simulink model "powertrain"  (R2026a)
settings: Solver=VariableStepAuto  StopTime=0.5  FixedStep=1/20e3  MaxStep=1e-5
PreLoadFcn:
  | try, p = fileparts(which(bdroot)); addpath(fullfile(p,'..', 'scripts')); addpath(fullfile(p,'..', 'models')); addpath(p); catch, end; init;
InitFcn:
  | try, p = fileparts(which(bdroot)); addpath(fullfile(p,'..', 'scripts')); addpath(fullfile(p,'..', 'models')); addpath(p); catch, end; init;
libraries: mcbcontrolslib x1
settings Model: Creator=probst  LastModifiedBy=niklasprobst
settings DebuggingCC: ParameterPrecisionLossMsg=none

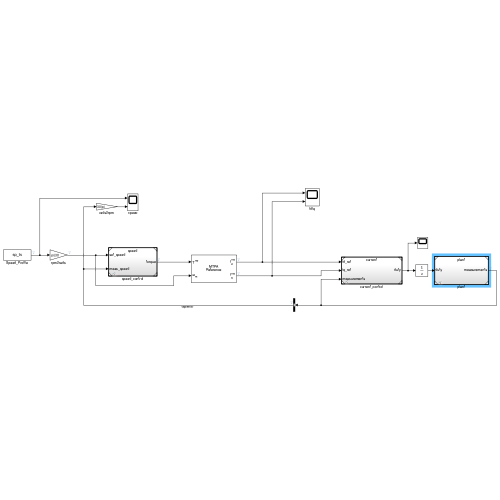
[thumbnail: Simulink's stored preview of the top-level diagram]
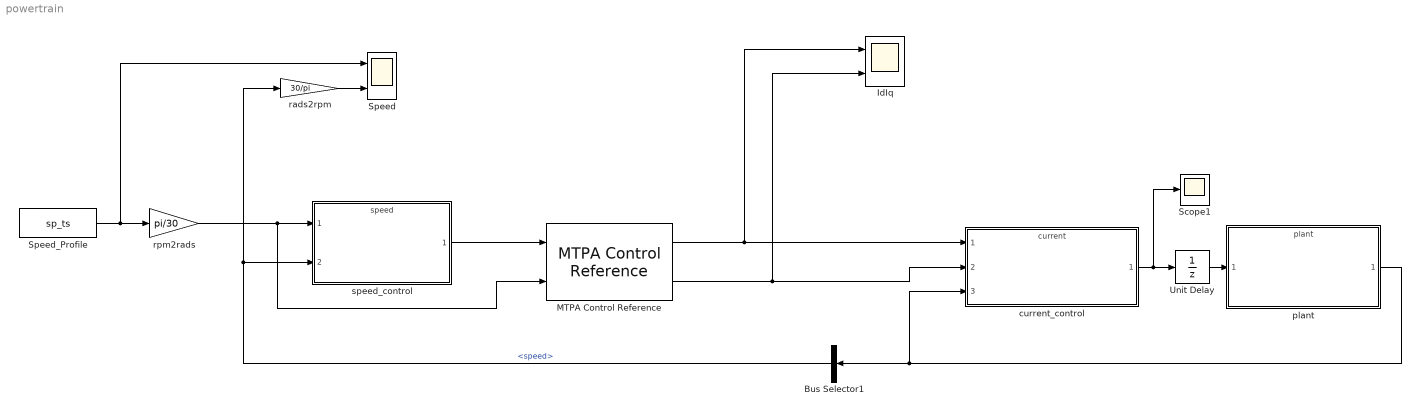
== system powertrain ==
  Bus Selector1 : BusSelector  OutputSignals=speed
  IdIq : Scope  NumInputPorts=2
      settings: ActiveDisplayYMinimum=-1  ActiveDisplayYMaximum=1
  MTPA Control Reference : mcbcontrolslib/MTPA Control Reference  VariantSelect=Interior PMSM  polePairs=pmsm.P  Rs=pmsm.Rs  Ld=pmsm.Ld  Lq=pmsm.Lq  FluxPM=pmsm.fl  ilimit=pmsm.I_rated  Vdc_input_select=Specify via dialog  V_dc=pmsm.V_rated  Units=SI Units  N_base=pmsm.N_base  I_base=19.3  T_base=1  V_base=24/sqrt(3)  N_base_disp=3182  MTPAiterator=on  iterCount=10
  Scope1 : Scope
      settings: ActiveDisplayYMinimum=0.45374474439973855  ActiveDisplayYMaximum=0.54625525560026145
  Speed : Scope  NumInputPorts=2
      settings: ActiveDisplayYMinimum=-2805.3468223093264  ActiveDisplayYMaximum=25248.121400783941
  Speed_Profile : FromWorkspace  VariableName=sp_ts
  Unit Delay : UnitDelay  SampleTime=-1
  current_control : ModelReference  ModelNameDialog=current.slx  SimulationMode=Normal  ModelReferenceVersion=1.91
  plant : ModelReference  ModelNameDialog=plant.slx  SimulationMode=Normal  ModelReferenceVersion=1.48
  rads2rpm : Gain  Gain=30/pi
  rpm2rads : Gain  Gain=pi/30
  speed_control : ModelReference  ModelNameDialog=speed.slx  SimulationMode=Normal  ModelReferenceVersion=1.38
  wires:
  Speed_Profile/1 -> rpm2rads/1, Speed/1
  rpm2rads/1 -> speed_control/1, MTPA Control Reference/2
  MTPA Control Reference/1 -> current_control/1, IdIq/1
  MTPA Control Reference/2 -> current_control/2, IdIq/2
  current_control/1 -> Unit Delay/1, Scope1/1
  Unit Delay/1 -> plant/1
  plant/1 -> current_control/3, Bus Selector1/1
  Bus Selector1/1 -> speed_control/2, rads2rpm/1  "<speed>"
  rads2rpm/1 -> Speed/2
  speed_control/1 -> MTPA Control Reference/1
